simulink model "modelo_diagrama_simulacion"  (R2015b)
settings: Solver=VariableStepAuto  StartTime=0.0  StopTime=10.0  RelTol=1e-3
undefined symbols (not defined in the file): G, Ts
settings Model: Creator=n221  LastModifiedBy=n221

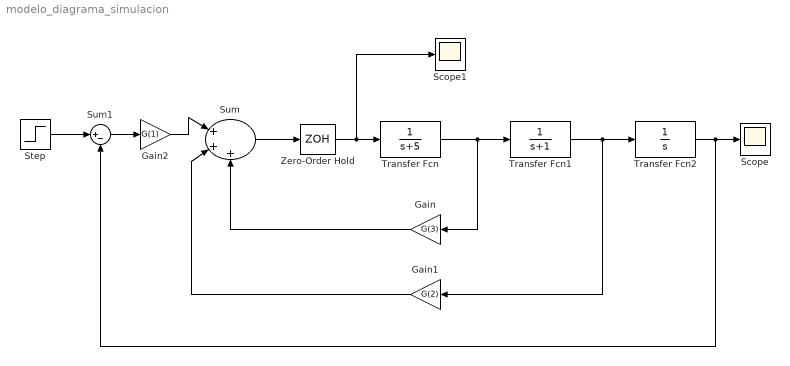
== system modelo_diagrama_simulacion ==
  Gain : Gain  Gain=G(3)
  Gain1 : Gain  Gain=G(2)
  Gain2 : Gain  Gain=G(1)
  Scope : Scope
  Scope1 : Scope
  Step : Step  SampleTime=0
  Sum : Sum  Inputs=|+++
  Sum1 : Sum  Inputs=|+-
  Transfer Fcn : TransferFcn  Denominator=[1 5]
  Transfer Fcn1 : TransferFcn  Denominator=[1 1]
  Transfer Fcn2 : TransferFcn  Denominator=[1 0]
  Zero-Order Hold : ZeroOrderHold  SampleTime=Ts
  wires:
  Transfer Fcn1/1 -> Gain1/1, Transfer Fcn2/1
  Transfer Fcn/1 -> Gain/1, Transfer Fcn1/1
  Zero-Order Hold/1 -> Scope1/1, Transfer Fcn/1
  Sum/1 -> Zero-Order Hold/1
  Step/1 -> Sum1/1
  Sum1/1 -> Gain2/1
  Transfer Fcn2/1 -> Sum1/2, Scope/1
  Gain2/1 -> Sum/1
  Gain/1 -> Sum/3
  Gain1/1 -> Sum/2
